simulink model "SimpleModel"  (R2019a)
settings: Solver=VariableStepAuto  StartTime=0.0  StopTime=10.0  RelTol=1e-3
settings Model: Creator=leand  LastModifiedBy=leand

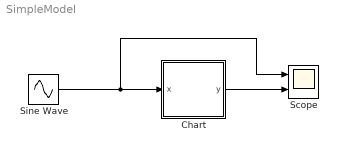
== system SimpleModel ==
  Chart : Stateflow chart  BlockKeywords=__PRM__SERIALIZED__DATA__:Stateflow Chart,Stateflow Diagram  TreatAsAtomicUnit=on
  Scope : Scope  NumInputPorts=2
  Sine Wave : Sin  SampleTime=0
  wires:
  Sine Wave/1 -> Scope/1, Chart/1(x)
  Chart/1(y) -> Scope/2

== stateflow chart SimpleModel/Chart ==
  note: https://www.mathworks.com/help/stateflow/gs/stateflow-charts.html
  note: Opção 1
  state ON [commented out]
    y=x;
  state OFF [commented out]
    y=0;
  note: Opção 2
  (default) -> ON [commented out]
  ON -> OFF [commented out] : [x<t0]
  OFF -> ON [commented out] : [x>=t0]
  (default) -> (junction 14)
  (junction 14) -> (junction 20) [order 2] : [x<t0]
  (junction 14) -> (junction 18) [order 1]
  (junction 20) -> (junction 23) : {y=0}
  (junction 18) -> (junction 25) : [x>=0]
  (junction 25) -> (junction 27) : {y=x}
  (junction 23) -> (junction 27)
  (junction 27) -> (junction 31)
  data: x input; y output; t0 constant double =0
